simulink model "Servomecanismo_LQR_lateral"  (R2018b)
settings: Solver=VariableStepAuto  StartTime=0.0  StopTime=500  RelTol=1e-3
values from neighbouring files (symbols this model uses):
  A = [xu,        xw*u0,         -u0*tan(aa0), -g*cos(tt0),     0 ... (first row only)    [long_ctes.m]    (also in modelo_L13_PD_lateral.m = [ybb yp+w0/u0 yr-1 g*cos(tt0)/u0 ; lbb lp lr 0 ; nbb np nr 0; real_servo_c_lateral.m = [ybb yp+w0/u0 yr-1 g*cos(tt0)/u0 0; lbb lp lr 0 0; nbb np nr)
  B = [xde,         xdf ... (first row only)    [long_ctes.m]    (also in modelo_L13_PD_lateral.m = [0 Ydr ; Lda Ldr ; Nda Ndr ; 0 0]; real_servo_c_lateral.m = [0 Ydr ; Lda Ldr ; Nda Ndr ; 0 0 ; 0 0])
  C = eye(4)    [modelo_L13_PD_lateral.m]    (also in real_servo_c_lateral.m = eye(5))
  Cc = C(2:1:4,:)    [real_servo_c_lateral.m]
  Cy = C(1:4:5,:)    [real_servo_c_lateral.m]
  D = [0 0; 0 0; 0 0; 0 0]    [modelo_L13_PD_lateral.m]    (also in real_servo_c_lateral.m = [0 0; 0 0; 0 0; 0 0; 0 0])
  deg = pi/180    (= 0.0174532925199)    [lateral_ctes.m]    (also in long_ctes.m; modelo_L13_PD_lateral.m; real_servo_c_lateral.m)
  Kc = [-0.0196 1.6622 -0.8045 -3.0813 -0.0000 0.9333]    [long_ctes.m]    (also in real_servo_c_lateral.m = k(:,2:1:4))
  Ky = k(:,1:4:5)    [real_servo_c_lateral.m]
libraries: simulink x3
settings Model: Creator=pedro  LastModifiedBy=Admin

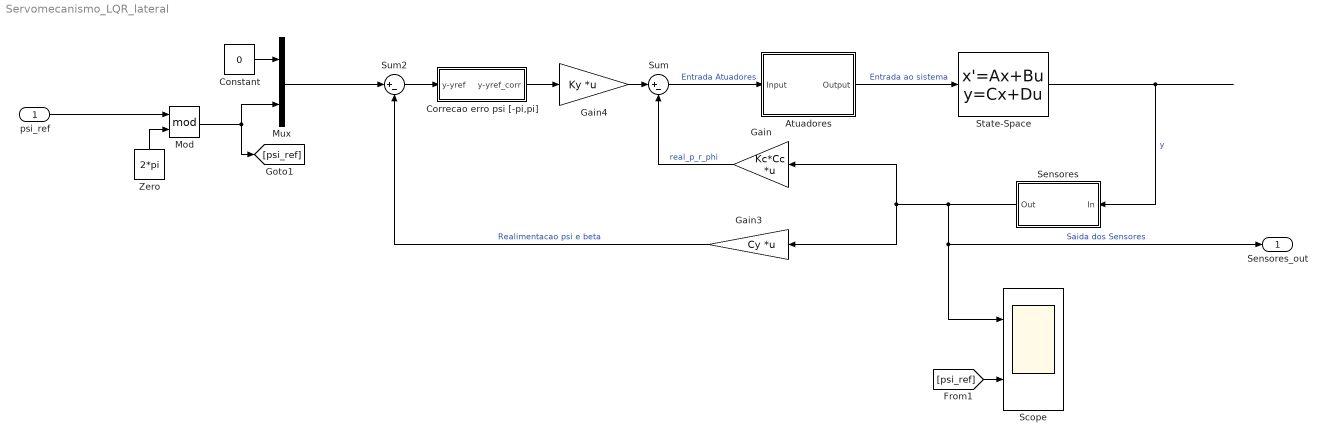
== system Servomecanismo_LQR_lateral ==
  psi_ref : Inport
  Atuadores : Subsystem
  Constant : Constant  Value=0
  Correcao erro psi [-pi,pi] : Subsystem
  Gain : Gain  Gain=Kc*Cc  Multiplication=Matrix(K*u)
  Gain3 : Gain  Gain=Cy  Multiplication=Matrix(K*u)
  Gain4 : Gain  Gain=Ky  Multiplication=Matrix(K*u)
  Mod : Math  Operator=mod  SaturateOnIntegerOverflow=on
  Mux : Mux  Inputs=2
  Scope : Scope  NumInputPorts=2
  Sensores : Subsystem
  State-Space : StateSpace  A=A  B=B  C=C  D=D  InitialCondition=0  ContinuousStateAttributes={'beta','p','r','pranchamento','guinada'}
  Sum : Sum  Inputs=|+-
  Sum2 : Sum  Inputs=|+-
  Zero : Constant  Value=2*pi  OutDataTypeStr=Inherit: Inherit via back propagation
  Sensores_out : Outport
  wires:
  Gain/1 -> Sum/2  "real_p_r_phi"
  Gain3/1 -> Sum2/2  "Realimentacao psi e beta"
  Mux/1 -> Sum2/1
  State-Space/1 -> Sensores/1(In)  "y"
  Gain4/1 -> Sum/1
  Sensores/1(Out) -> Gain/1, Gain3/1, Scope/1, Sensores_out/1  "Saida dos Sensores"
  Sum/1 -> Atuadores/1(Input)  "Entrada Atuadores"
  Atuadores/1(Output) -> State-Space/1  "Entrada ao sistema"
  Mod/1 -> Mux/2, [psi_ref]
  Zero/1 -> Mod/2
  Correcao erro psi [-pi,pi]/1(y-yref_corr) -> Gain4/1
  Sum2/1 -> Correcao erro psi [-pi,pi]/1(y-yref)
  Constant/1 -> Mux/1
  psi_ref/1 -> Mod/1
  [psi_ref] -> Scope/2

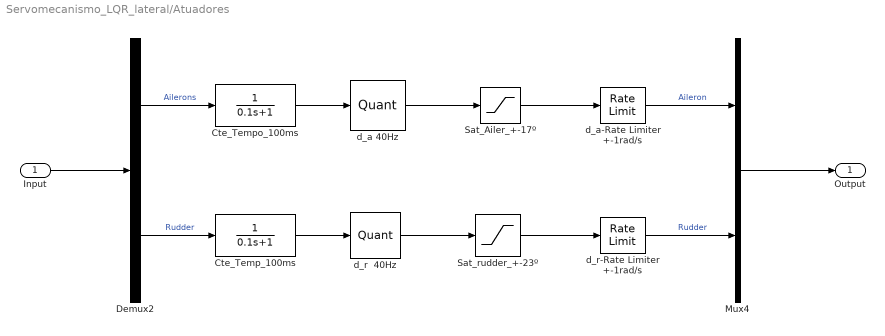
== system Servomecanismo_LQR_lateral/Atuadores ==
  Input : Inport
  Cte_Temp_100ms : TransferFcn  Denominator=[0.1 1]
  Cte_Tempo_100ms : TransferFcn  Denominator=[0.1 1]
  Demux2 : Demux  Outputs=2
  Mux4 : Mux  Inputs=2
  Sat_Ailer_+-17º : Saturate  UpperLimit=17*deg  LowerLimit=-17*deg
  Sat_rudder_+-23º : Saturate  UpperLimit=23*deg  LowerLimit=-23*deg
  d_a 40Hz : Quantizer  QuantizationInterval=1/40
  d_a-Rate Limiter +-1rad/s : RateLimiter  SampleTimeMode=inherited
  d_r  40Hz : Quantizer  QuantizationInterval=1/40
  d_r-Rate Limiter +-1rad/s : RateLimiter  SampleTimeMode=inherited
  Output : Outport
  wires:
  d_a 40Hz/1 -> Sat_Ailer_+-17º/1
  Input/1 -> Demux2/1
  Sat_rudder_+-23º/1 -> d_r-Rate Limiter +-1rad/s/1
  Mux4/1 -> Output/1
  Cte_Temp_100ms/1 -> d_r  40Hz/1
  d_r  40Hz/1 -> Sat_rudder_+-23º/1
  d_r-Rate Limiter +-1rad/s/1 -> Mux4/2  "Rudder"
  Demux2/2 -> Cte_Temp_100ms/1  "Rudder"
  d_a-Rate Limiter +-1rad/s/1 -> Mux4/1  "Aileron"
  Demux2/1 -> Cte_Tempo_100ms/1  "Ailerons"
  Cte_Tempo_100ms/1 -> d_a 40Hz/1
  Sat_Ailer_+-17º/1 -> d_a-Rate Limiter +-1rad/s/1

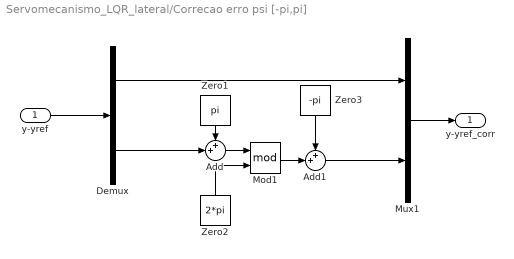
== system Servomecanismo_LQR_lateral/Correcao erro psi [-pi,pi] ==
  y-yref : Inport
  Add : Sum  Inputs=++|
  Add1 : Sum  Inputs=++|
  Demux : Demux  Outputs=2
  Mod1 : Math  Operator=mod  SaturateOnIntegerOverflow=on
  Mux1 : Mux  Inputs=2
  Zero1 : Constant  Value=pi  OutDataTypeStr=Inherit: Inherit via back propagation
  Zero2 : Constant  Value=2*pi  OutDataTypeStr=Inherit: Inherit via back propagation
  Zero3 : Constant  Value=-pi  OutDataTypeStr=Inherit: Inherit via back propagation
  y-yref_corr : Outport
  wires:
  Zero1/1 -> Add/1
  Zero3/1 -> Add1/1
  Zero2/1 -> Mod1/2
  Mod1/1 -> Add1/2
  y-yref/1 -> Demux/1
  Add/1 -> Mod1/1
  Mux1/1 -> y-yref_corr/1
  Add1/1 -> Mux1/2
  Demux/2 -> Add/2
  Demux/1 -> Mux1/1

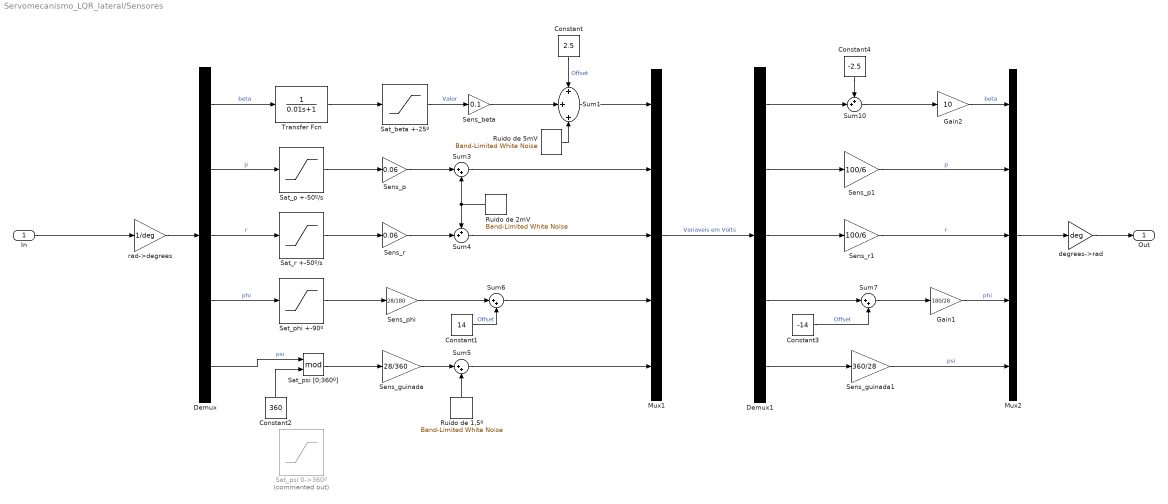
== system Servomecanismo_LQR_lateral/Sensores ==
  In : Inport
  Constant : Constant  Value=2.5
  Constant1 : Constant  Value=14
  Constant2 : Constant  Value=360
  Constant3 : Constant  Value=-14
  Constant4 : Constant  Value=-2.5
  Demux : Demux  Outputs=5
  Demux1 : Demux  Outputs=5
  Gain1 : Gain  Gain=180/28
  Gain2 : Gain  Gain=10
  Mux1 : Mux  Inputs=5
  Mux2 : Mux  Inputs=5
  Ruido de 1,5º : simulink/Sources/Band-Limited White Noise  Cov=[(1.5*28/360)^2/40]  Ts=1/40  seed=[23341]
  Ruido de 2mV : simulink/Sources/Band-Limited White Noise  Cov=[(0.002)^2/40]  Ts=1/40  seed=[23341]
  Ruido de 5mV : simulink/Sources/Band-Limited White Noise  Cov=[(0.005)^2/40]  Ts=1/40  seed=[23341]
  Sat_beta +-25º : Saturate  UpperLimit=+25  LowerLimit=-25
  Sat_p +-50º/s : Saturate  UpperLimit=+50  LowerLimit=-50
  Sat_phi +-90º : Saturate  UpperLimit=+90  LowerLimit=-90
  Sat_psi 0->360º : Saturate  Commented=on  UpperLimit=360  LowerLimit=-360
  Sat_psi [0;360º] : Math  Operator=mod  SaturateOnIntegerOverflow=on
  Sat_r +-50º/s : Saturate  UpperLimit=+50  LowerLimit=-50
  Sens_beta : Gain  Gain=0.1
  Sens_guinada : Gain  Gain=28/360
  Sens_guinada1 : Gain  Gain=360/28
  Sens_p : Gain  Gain=0.06
  Sens_p1 : Gain  Gain=100/6
  Sens_phi : Gain  Gain=28/180
  Sens_r : Gain  Gain=0.06
  Sens_r1 : Gain  Gain=100/6
  Sum1 : Sum  Inputs=+++
  Sum10 : Sum  Inputs=++|
  Sum{3,5..7} (4 alike) : Sum  Inputs=|++
  Sum4 : Sum  Inputs=++|
  Transfer Fcn : TransferFcn  Denominator=[0.01 1]
  degrees->rad : Gain  Gain=deg
  rad->degrees : Gain  Gain=1/deg
  Out : Outport
  wires:
  Sens_guinada/1 -> Sum5/1
  Demux1/4 -> Sum7/1
  Gain2/1 -> Mux2/1  "beta"
  Sens_phi/1 -> Sum6/1
  Demux1/5 -> Sens_guinada1/1
  Sat_p +-50º/s/1 -> Sens_p/1
  Sum6/1 -> Mux1/4
  Sens_p1/1 -> Mux2/2  "p"
  Constant1/1 -> Sum6/2  "Offset"
  Sens_beta/1 -> Sum1/2
  Ruido de 5mV/1 -> Sum1/3
  Sens_r1/1 -> Mux2/3  "r"
  In/1 -> rad->degrees/1
  Sat_beta +-25º/1 -> Sens_beta/1  "Valor"
  Constant3/1 -> Sum7/2  "Offset"
  degrees->rad/1 -> Out/1
  Sum4/1 -> Mux1/3
  Demux/4 -> Sat_phi +-90º/1  "phi"
  Sum7/1 -> Gain1/1
  Sens_r/1 -> Sum4/2
  Sum10/1 -> Gain2/1
  Gain1/1 -> Mux2/4  "phi"
  rad->degrees/1 -> Demux/1
  Mux1/1 -> Demux1/1  "Variaveis em Volts"
  Sens_guinada1/1 -> Mux2/5  "psi"
  Sum5/1 -> Mux1/5
  Sat_phi +-90º/1 -> Sens_phi/1
  Demux/2 -> Sat_p +-50º/s/1  "p"
  Sum1/1 -> Mux1/1
  Demux/3 -> Sat_r +-50º/s/1  "r"
  Ruido de 1,5º/1 -> Sum5/2
  Ruido de 2mV/1 -> Sum3/2, Sum4/1
  Mux2/1 -> degrees->rad/1
  Sens_p/1 -> Sum3/1
  Sum3/1 -> Mux1/2
  Constant/1 -> Sum1/1  "Offset"
  Sat_r +-50º/s/1 -> Sens_r/1
  Demux1/3 -> Sens_r1/1
  Demux1/2 -> Sens_p1/1
  Demux/1 -> Transfer Fcn/1  "beta"
  Transfer Fcn/1 -> Sat_beta +-25º/1
  Demux1/1 -> Sum10/2
  Constant4/1 -> Sum10/1
  Demux/5 -> Sat_psi [0;360º]/1  "psi"
  Sat_psi [0;360º]/1 -> Sens_guinada/1
  Constant2/1 -> Sat_psi [0;360º]/2
